simulink model "BMS_Harness_ContactorMgmt"  (R2024a)
settings: configuration reference "AutosarConfig" (kept outside this file)
libraries: SignalEditorBlockLib x1
settings Model: DataDictionary=BMS_Software_DD.sldd  Creator=smuckati  LastModifiedBy=smuckati
settings ConfigSetRef: SourceName=AutosarConfig

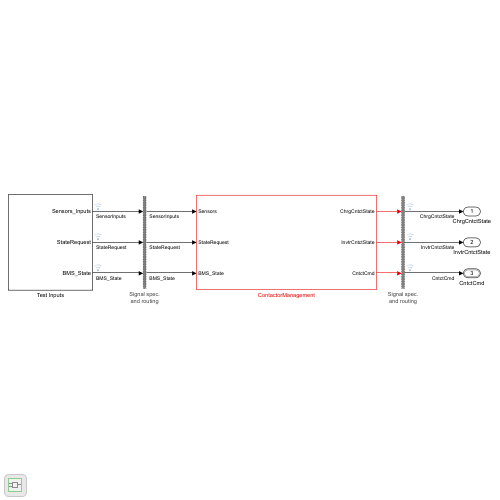
[thumbnail: Simulink's stored preview of the top-level diagram]
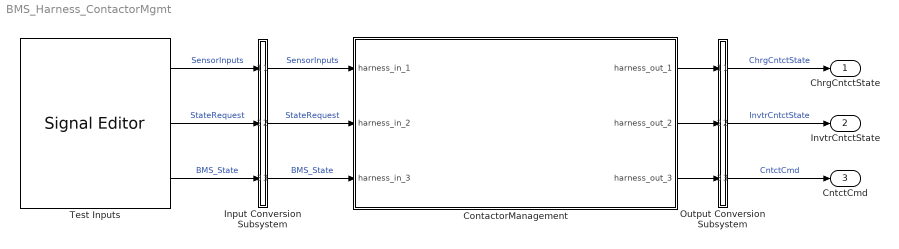
== system BMS_Harness_ContactorMgmt ==
  ContactorManagement : Subsystem  Tag=__SL_testing_harness_stub_
  Input Conversion Subsystem : Subsystem  Tag=__SLT_ICS__  Description=|
      | Signal spec.
      | and routing
      settings: AttributesFormatString=%<Description>
  Output Conversion Subsystem : Subsystem  Tag=__SLT_OCS__  Description=|
      | Signal spec.
      | and routing
      settings: AttributesFormatString=%<Description>
  Test Inputs : SignalEditorBlockLib/Signal Editor  FileName=ContactorMgmt_HarnessInputs.mat  ActiveScenario=Charging  ActiveSignal=Sensors_Inputs  IsBus=on  OutputBusObjectStr=Bus: Sensors  SampleTime=0.1  Interpolate=off  ZeroCross=off  OutputAfterFinalValue=Setting to zero  Unit=inherit  PreserveSignalName=on  ApplySigPropsToAllScenarios=on  ApplySigPropsToAllSignals=off
  ChrgCntctState : Outport
  InvtrCntctState : Outport  Port=2
  CntctCmd : Outport  Port=3  OutDataTypeStr=Bus: CntctCmd
  wires:
  Test Inputs/1 -> Input Conversion Subsystem/1(Inport_1)  "SensorInputs"
  Test Inputs/2 -> Input Conversion Subsystem/2(Inport_2)  "StateRequest"
  Test Inputs/3 -> Input Conversion Subsystem/3(Inport_3)  "BMS_State"
  Output Conversion Subsystem/1(Outport_1) -> ChrgCntctState/1  "ChrgCntctState"
  Output Conversion Subsystem/2(Outport_2) -> InvtrCntctState/1  "InvtrCntctState"
  Output Conversion Subsystem/3(Outport_3) -> CntctCmd/1  "CntctCmd"
  Input Conversion Subsystem/1(Outport_1) -> ContactorManagement/1(harness_in_1)  "SensorInputs"
  Input Conversion Subsystem/2(Outport_2) -> ContactorManagement/2(harness_in_2)  "StateRequest"
  Input Conversion Subsystem/3(Outport_3) -> ContactorManagement/3(harness_in_3)  "BMS_State"
  ContactorManagement/1(harness_out_1) -> Output Conversion Subsystem/1(Inport_1)
  ContactorManagement/2(harness_out_2) -> Output Conversion Subsystem/2(Inport_2)
  ContactorManagement/3(harness_out_3) -> Output Conversion Subsystem/3(Inport_3)

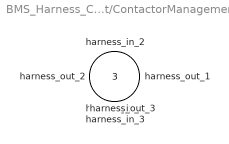
== system BMS_Harness_ContactorMgmt/ContactorManagement ==
  harness_in_1 : Inport
  harness_in_2 : Inport  Port=2
  harness_in_3 : Inport  Port=3
  harness_out_1 : Outport
  harness_out_2 : Outport  Port=2
  harness_out_3 : Outport  Port=3

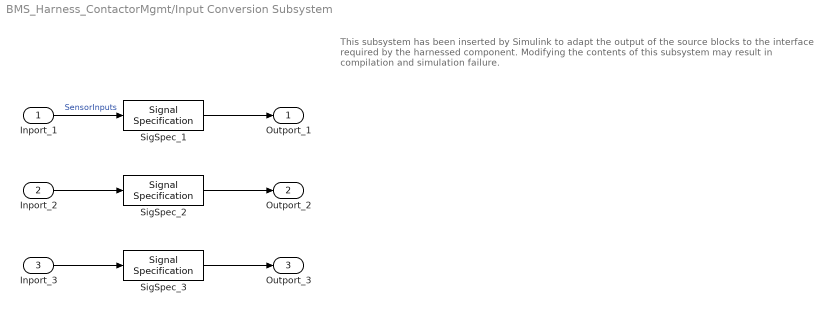
== system BMS_Harness_ContactorMgmt/Input Conversion Subsystem ==
  note: This subsystem has been inserted by Simulink to adapt the output of the source blocks to the interface required by the harnessed component.
      |  Modifying the contents of this subsystem may result in compilation and simulation failure.
  Inport_1 : Inport
  Inport_2 : Inport  Port=2
  Inport_3 : Inport  Port=3
  SigSpec_1 : SignalSpecification  OutDataTypeStr=Bus: Sensors  Dimensions=[1]  SampleTime=0.1  BusOutputAsStruct=on
  SigSpec_2 : SignalSpecification  OutDataTypeStr=Enum: SRE  Dimensions=[1]  SampleTime=0.1
  SigSpec_3 : SignalSpecification  OutDataTypeStr=Enum: BMS_State_Enum  Dimensions=[1]  SampleTime=0.1
  Outport_1 : Outport
  Outport_2 : Outport  Port=2
  Outport_3 : Outport  Port=3
  wires:
  SigSpec_1/1 -> Outport_1/1
  Inport_1/1 -> SigSpec_1/1  "SensorInputs"
  SigSpec_2/1 -> Outport_2/1
  Inport_2/1 -> SigSpec_2/1
  SigSpec_3/1 -> Outport_3/1
  Inport_3/1 -> SigSpec_3/1

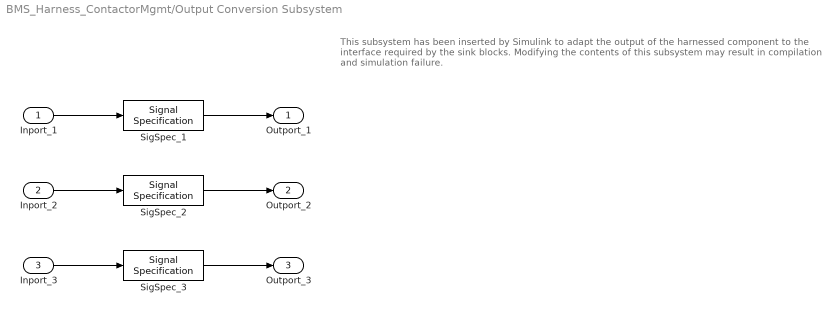
== system BMS_Harness_ContactorMgmt/Output Conversion Subsystem ==
  note: This subsystem has been inserted by Simulink to adapt the output of the harnessed component to the interface required by the sink blocks.
      |  Modifying the contents of this subsystem may result in compilation and simulation failure.
  Inport_1 : Inport
  Inport_2 : Inport  Port=2
  Inport_3 : Inport  Port=3
  SigSpec_1 : SignalSpecification  OutDataTypeStr=Enum: Contact  Dimensions=[1]  SampleTime=0.1
  SigSpec_2 : SignalSpecification  OutDataTypeStr=Enum: Contact  Dimensions=[1]  SampleTime=0.1
  SigSpec_3 : SignalSpecification  OutDataTypeStr=Bus: CntctCmd  Dimensions=[1]  SampleTime=0.1  BusOutputAsStruct=on
  Outport_1 : Outport
  Outport_2 : Outport  Port=2
  Outport_3 : Outport  Port=3
  wires:
  Inport_1/1 -> SigSpec_1/1
  SigSpec_1/1 -> Outport_1/1
  Inport_2/1 -> SigSpec_2/1
  SigSpec_2/1 -> Outport_2/1
  Inport_3/1 -> SigSpec_3/1
  SigSpec_3/1 -> Outport_3/1
